simulink model "Target_Control_System"  (R2021b)
settings: Solver=FixedStepDiscrete  StartTime=0.0  StopTime=5  RelTol=1e-3
PreLoadFcn:
  | RTWConfigurationCB('preloadfcn', bdroot);
PostLoadFcn:
  | load('configuration/data_struct.mat');
  | load('configuration/fluxMaps_propMotor.mat');
  | load('configuration/parameterInit_PROP.mat');
  | load('configuration/parameterInit_PUMP.mat');
  | load('configuration/parameterInit_PITCH.mat');
  | load('configuration/parameterInit_TILT.mat');
  | %load('configuration/base_workspace_signal_definition.mat');
  | %load('resolvedatastores_to_baseworkspace_for_faster_simulation.mat');
model workspace (MAT data in the model file):
  SIMULATION_OPTIONS : Simulink.Parameter (value not decoded)
  TARGET_CODE_GEN : Simulink.Parameter (value not decoded)
  TCS_SAMPLE_FREQ_HZ : Simulink.Parameter (value not decoded)
symbols that are objects in the model workspace (value not decoded): TARGET_CODE_GEN, TCS_SAMPLE_FREQ_HZ
undefined symbols (not defined in the file): A_DQ_REF_LPF_INIT__PITCH, A_DQ_REF_LPF_INIT__PROP, A_DQ_REF_LPF_INIT__PUMP, A_DQ_REF_LPF_INIT__TILT, A_OBSERVER_CONFIDENCE_INIT__PITCH, A_OBSERVER_CONFIDENCE_INIT__PROP, A_OBSERVER_CONFIDENCE_INIT__PUMP, A_OBSERVER_CONFIDENCE_INIT__TILT, ACTUATOR_MAX_ANGLE_TRIP__PITCH, ACTUATOR_MIN_ANGLE_TRIP__PITCH, ACTUATOR_POS_SENSOR_INV_DIRECTION__PITCH, ACTUATOR_POS_SENSOR_INV_DIRECTION__TILT, ACTUATOR_POS_SENSOR_OFFSET__PITCH, ACTUATOR_POS_SENSOR_OFFSET__TILT, ADC_scaler1_baseaddr_TILT, ADC_SCALER_FLOAT_TO_FIXPOINT_EXPANSION, ANGLE_ELEC_FROM_SENSOR_OFFSET_INIT__PITCH, ANGLE_ELEC_FROM_SENSOR_OFFSET_INIT__PROP, ANGLE_ELEC_FROM_SENSOR_OFFSET_INIT__PUMP, ANGLE_ELEC_FROM_SENSOR_OFFSET_INIT__TILT, AUTO_CLEAR_FAULTS_ENABLED__PITCH, AUTO_CLEAR_FAULTS_ENABLED__PROP, AUTO_CLEAR_FAULTS_ENABLED__PUMP, AUTO_CLEAR_FAULTS_ENABLED__TILT, AUTO_CLEAR_FAULTS_WAIT_TICKS__PITCH, AUTO_CLEAR_FAULTS_WAIT_TICKS__PROP, AUTO_CLEAR_FAULTS_WAIT_TICKS__PUMP, AUTO_CLEAR_FAULTS_WAIT_TICKS__TILT, AUTO_I_ZERO_IDLE_TICKS__PITCH, AUTO_I_ZERO_IDLE_TICKS__PROP, AUTO_I_ZERO_IDLE_TICKS__PUMP, AUTO_I_ZERO_IDLE_TICKS__TILT, AUTO_I_ZERO_OFFSET_IDC_THRESHOLD__PITCH, AUTO_I_ZERO_OFFSET_IDC_THRESHOLD__PROP, AUTO_I_ZERO_OFFSET_IDC_THRESHOLD__PUMP, AUTO_I_ZERO_OFFSET_IDC_THRESHOLD__TILT, AUTO_I_ZERO_OFFSET_IPH_THRESHOLD__PITCH, AUTO_I_ZERO_OFFSET_IPH_THRESHOLD__PROP, AUTO_I_ZERO_OFFSET_IPH_THRESHOLD__PUMP, AUTO_I_ZERO_OFFSET_IPH_THRESHOLD__TILT, AUTO_SENSORLESS_SWITCHOVER_DISABLE_OMEGA, AUTO_SENSORLESS_SWITCHOVER_ENABLE_OMEGA, AUTO_SENSORLESS_SWITCHOVER_MIN_CONFIDENCE, AUXILIARY_PROTECTION_UNIT_BASEADDR__TILT, blanking_max_error_omega_INIT_PITCH, blanking_max_error_omega_INIT_TILT, blanking_max_error_position_INIT_PITCH, blanking_max_error_position_INIT_TILT, BRUTE_START_I_Q_REF_RAMP_SPEED__PITCH, BRUTE_START_I_Q_REF_RAMP_SPEED__PROP, BRUTE_START_I_Q_REF_RAMP_SPEED__PUMP, BRUTE_START_I_Q_REF_RAMP_SPEED__TILT, CONTROL_LOOP_DT_INIT__PITCH, CONTROL_LOOP_DT_INIT__PROP, CONTROL_LOOP_DT_INIT__PUMP, CONTROL_LOOP_DT_INIT__TILT, CORRECTION_FILTER_SCALE__PITCH, CORRECTION_FILTER_SCALE__PROP, CORRECTION_FILTER_SCALE__PUMP, CORRECTION_FILTER_SCALE__TILT ... (+458)
libraries: simulink x178, Reusables_Lib x24
(part 47 of 47)

== stateflow chart Target_Control_System/MainLoop/propMotor_mainLoop/motorTaskMainFastStep(&oProp)/enableDrive(&oProp) ==
  state Disabled
    state Default
    state Disable_Drive
      entry:
      oProp.oMot_.oState_.uiDriveState_ = 100;
      oProp.oMot_.oOut_.uiEnableGateDrive_ = 0x0;
      oProp.oMot_.oOut_.uiCurrentControllerActive_ = 0;
    state Simulation
      entry:
      oProp.oMot_.oState_.uiDriveState_ = 101;
      oProp.oMot_.oOut_.uiEnableGateDrive_ = 0x0;
    (default) -> (junction 391)
    (junction 391) -> Default [order 3]
    (junction 391) -> Disable_Drive [order 2] : [oProp.oMot_.oState_.uiDriveState_ >= 200 && ....
        |  oProp.oMot_.oState_.uiDriveState_ <= 299]
    (junction 391) -> Simulation [order 1] : [TARGET_CODE_GEN ==0]
  state Position_hold_mode
    // Mostly intended for the VP. In position hold mode, the inverter will inject 0 RPM current in the motor to passively hold a motor in place.
    // The position sensors are not needed for this.
    // When issuing the enable command, the drive enters state 226, which is just for flagging, the inverters do not actually turn on.
    // (Use a special command for that.)
    entry:
    oProp.oMot_.oState_.uiDriveState_ = 226;
    oProp.oIsr_.oParam_.oPiDataIq_.fState_ = 0;
    oProp.oIsr_.oParam_.oPiDataId_.fState_ = 0;
    // Pre-set 50% duty
    oProp.oMot_.oOut_.uiPwmRequestFromMain_ = 1;
    oProp.oMot_.oOut_.uiPwmDutyTicksFromMainA_ = uint32((oProp.oMot_.oParam_.fPwmPeriodTicksMainloopFloat_)/2);
    oProp.oMot_.oOut_.uiPwmDutyTicksFromMainB_ = uint32((oProp.oMot_.oParam_.fPwmPeriodTicksMainloopFloat_)/2);
    oProp.oMot_.oOut_.uiPwmDutyTicksFromMainC_ = uint32((oProp.oMot_.oParam_.fPwmPeriodTicksMainloopFloat_)/2);
  state DC_undervoltage_trip
    state Fault_A
      entry:
      oProp.oMot_.oOut_.uiCurrentControllerActive_ = 0;
      oProp.oMot_.oOut_.uiEnableGateDrive_ = 0;
    state Fault_B
      // If we were already in a fault state, store the previous fault:
      entry:
      oProp.oMot_.oOut_.uiLastFaultState_ = oProp.oMot_.oState_.uiDriveState_;
    state Fault_C
      entry:
      oProp.oMot_.oState_.uiDriveState_ = 1003;
    (default) -> (junction 164)
    (junction 164) -> Fault_A [order 1] : [oProp.oMot_.oState_.uiDriveState_>= 200]
    (junction 164) -> Fault_C [order 3]
    (junction 164) -> Fault_B [order 2] : [oProp.oMot_.oState_.uiDriveState_>= 1000]
    Fault_A -> Fault_B [order 1] : [oProp.oMot_.oState_.uiDriveState_>= 1000]
    Fault_A -> Fault_C [order 2]
    Fault_B -> Fault_C
  state Slave_start
    // Slave start is not applicable to position control.
    // Not a position control inverter; slave role is set: Perform a slave start (wait for the motor to 'somehow' reach a minimum speed, then jump on).
    entry:
    // We have to set one item aside; the desired rotation direction, as signalled by the sign of the current
    oProp.oMot_.oState_.fForcedAngleStartDirection_ = single(oProp.oMot_.oIn_.fIqSetpoint_ >= 0);
    // Don't actually turn on the output stage, but instead, monitor the motor feedback.
    // Once confident, perform a running start.
    // The rest is handled via state machine.
    oProp.oMot_.oState_.uiDriveState_ = 220;
  state setupForFlyingStart
    entry:
    oProp.oMot_.oOut_.uiPwmDutyTicksFromMainA_ = uint32((oProp.oMot_.oParam_.fPwmPeriodTicksMainloopFloat_)/2);
    oProp.oMot_.oOut_.uiPwmDutyTicksFromMainB_ = uint32((oProp.oMot_.oParam_.fPwmPeriodTicksMainloopFloat_)/2);
    oProp.oMot_.oOut_.uiPwmDutyTicksFromMainC_ = uint32((oProp.oMot_.oParam_.fPwmPeriodTicksMainloopFloat_)/2);
    oProp.oMot_.oState_.oRampDataOmegaERef_.fRampOut_ = oProp.oMot_.oIn_.fOmegaEObserverLpf2_;
    oProp.oMot_.oState_.oRampDataIqRef_.fRampOut_ = 0.0;
    oProp.oIsr_.oParam_.oPiDataIq_.fState_ = 0.0F;
    oProp.oIsr_.oParam_.oPiDataId_.fState_ = 0.0F;
    oProp.oMot_.oParam_.oPiDataRpm_.fState_ = 0.0F;
    oProp.oMot_.oParam_.oPid2DataRpmCtrl_.fState_ = 0.0F;
    oProp.oMot_.oState_.uiDriveState_ = 200;
    oProp.oIsr_.oState_.fOverspeedProtectionScaler_ = 1.0;
    oProp.oMot_.oState_.oPosSensor_.iAngleElecFromSensorNumOfIdenticalValues_ = 0;
    // release gate signals
    oProp.oMot_.oOut_.uiEnableGateDrive_ = 0x7;
    // Release control in main interrupt
    oProp.oMot_.oOut_.uiCurrentControllerActive_ = 1;
    // [SZ]: add automatic fan control here
  state Enabled
    // [SZ]: Still need to model the setupForFlyingStart() function, which involves calling NEON sin/cos functions in Stateflow
    state Open_loop_start
      // Open loop start from standstill. Risky, and rough on hardware
      state Open_loop_start_A
        entry:
        oProp.oMot_.oState_.oRampDataFluxFeedforwardGain_.fRampOut_ = 0.0;
        oProp.oMot_.oState_.oRampDataOmegaERef_.fRampOut_ = 0.0;
        oProp.oMot_.oState_.oRampDataIqRef_.fRampOut_ = 0.0;
        oProp.oMot_.oState_.uiDriveState_ = 200;
      state Open_loop_start_B
        entry:
        oProp.oMot_.oState_.uiDriveState_ = 205;
      (default) -> Open_loop_start_A
      Open_loop_start_A -> Open_loop_start_B [order 1] : [oProp.oMot_.oParam_.uiAutomaticFanControlMode_ == 1]
    state Standing_start
      // ----- Set up for forced angle start ----
      state Store_reference
        // Store original references and ramp rates aside:
        entry:
        oProp.oMot_.oState_.fForcedAngleStartOrigIRamp_ = oProp.oMot_.oState_.oRampDataIqRef_.oParam_.fUpslope_;
        // TODO: whatabout downslope?
        oProp.oMot_.oState_.fForcedAngleStartOrigOmega_ = oProp.oMot_.oState_.oRampDataOmegaERef_.fSetpoint_;
        oProp.oMot_.oState_.fForcedAngleStartOrigOmegaRamp_ = oProp.oMot_.oState_.oRampDataOmegaERef_.oParam_.fUpslope_;
        // The downslope is never touched, as it doesn't matter for forced angle start
        oProp.oMot_.oState_.uiForcedAngleStartOrigSpeedControllerActive_ = oProp.oMot_.oState_.uiSpeedControllerActive_;
        // We have to set one item aside; the desired rotation direction, as signalled by the sign of the current
        oProp.oMot_.oState_.fForcedAngleStartDirection_ = single(oProp.oMot_.oIn_.fIqSetpoint_ >= 0);
      state Global_signal
        // Signals to the rest of the program.
        oProp.oMot_.oOut_.uiForcedAngle_ = 1;
        oProp.oMot_.oState_.uiDriveState_ = 211;
      state Initialization
        // Set up initial values
        entry:
        oProp.oMot_.oState_.fIqRefBeforeRamp_ = oProp.oMot_.oParam_.fForcedAngleIRef_;
        oProp.oMot_.oState_.oRampDataIqRef_.oParam_.fUpslope_ = oProp.oMot_.oParam_.fForcedAngleIRamp_*10*(TARGET_CODE_GEN==0)+...
        oProp.oMot_.oParam_.fForcedAngleIRamp_*(TARGET_CODE_GEN==1); // Adjust for 100 Hz state machine in the simulation mode
        oProp.oMot_.oState_.oRampDataIqRef_.oParam_.fDownslope_ = oProp.oMot_.oState_.oRampDataIqRef_.oParam_.fUpslope_;
        oProp.oMot_.oState_.oRampDataOmegaERef_.oParam_.fUpslope_ = oProp.oMot_.oParam_.fForcedAngleOmegaERamp_*10*(TARGET_CODE_GEN==0)+...
        oProp.oMot_.oParam_.fForcedAngleOmegaERamp_*(TARGET_CODE_GEN==1); // Adjust for 100 Hz state machine in the simulation mode
        oProp.oMot_.oState_.oRampDataOmegaERef_.fRampOut_ = 0.0F;
        oProp.oMot_.oState_.oRampDataOmegaERef_.fSetpoint_ = 0.0F;
        oProp.oMot_.oState_.oRampDataIqRef_.fRampOut_ = 0.0F;
        oProp.oMot_.oState_.uiSpeedControllerActive_ = 0;
        oProp.oMot_.oState_.uiForcedAngleStartParametersSet_ = 1;
        oProp.oMot_.oState_.oRampDataFluxFeedforwardGain_.fRampOut_ = 0.0F;
      (default) -> Global_signal
      Global_signal -> (junction 233)
      (junction 233) -> Store_reference [order 1] : [!(oProp.oMot_.oState_.uiForcedAngleStartParametersSet_ == 1)]
      (junction 233) -> Initialization [order 2]
      Store_reference -> Initialization
    state Half_duty_preset
      // Pre-set 50% duty
      entry:
      oProp.oMot_.oOut_.uiPwmRequestFromMain_ = 1;
      oProp.oMot_.oOut_.uiPwmDutyTicksFromMainA_ = uint32((oProp.oMot_.oParam_.fPwmPeriodTicksMainloopFloat_)/2);
      oProp.oMot_.oOut_.uiPwmDutyTicksFromMainB_ = uint32((oProp.oMot_.oParam_.fPwmPeriodTicksMainloopFloat_)/2);
      oProp.oMot_.oOut_.uiPwmDutyTicksFromMainC_ = uint32((oProp.oMot_.oParam_.fPwmPeriodTicksMainloopFloat_)/2);
      oProp.oIsr_.oParam_.oPiDataIq_.fState_ = 0.0F;
      oProp.oIsr_.oParam_.oPiDataId_.fState_ = 0.0F;
      oProp.oMot_.oParam_.oPiDataRpm_.fState_ = 0.0F;
      oProp.oMot_.oParam_.oPid2DataRpmCtrl_.fState_ = 0.0F;
      oProp.oMot_.oState_.oPosSensor_.oPidDataPosCtrl_.fState_ = 0.0F;
      oProp.oMot_.oState_.oRampDataPos_.fRampOut_ = oProp.oMot_.oState_.oPosSensor_.oGbx_.fCurrentOutputAngle_;
      // Prevent jerk motions on start up.
      // [SZ]: Moved here to avoid the "Unconditional Path Out of State with During Actions or Child States" warning
    state Release_gate_signal
      entry:
      oProp.oIsr_.oState_.fOverspeedProtectionScaler_ = 1.0;
      oProp.oMot_.oState_.oPosSensor_.iAngleElecFromSensorNumOfIdenticalValues_ = 0;
      // release gate signals
      oProp.oMot_.oOut_.uiEnableGateDrive_ = 0x7;
      oProp.oMot_.oOut_.uiCurrentControllerActive_ = 1; // Release control in main interrupt
    (default) -> (junction 184)
    (junction 184) -> Open_loop_start [order 2]
    (junction 184) -> Standing_start [order 1] : [oProp.oMot_.oState_.uiForcedAngleStart_ == 1]
    Open_loop_start_A -> Half_duty_preset [order 2]
    Open_loop_start_B -> Half_duty_preset
    Initialization -> Half_duty_preset
    Half_duty_preset -> Release_gate_signal
  (default) -> Disabled
  Slave_start -> Disabled : [!(oProp.oMot_.oOut_.uiEnable_ == 1)]
  Position_hold_mode -> Disabled : [!(oProp.oMot_.oOut_.uiEnable_ == 1)]
  (junction 192) -> Disabled [order 1] : [oProp.oMot_.oState_.uiDriveState_ < 101 || oProp.oMot_.oState_.uiDriveState_ > 104 || !(oProp.oMot_.oOut_.uiEnable_ == 1)]
  Disabled -> (junction 192) : [oProp.oMot_.oOut_.uiEnable_ == 1]
  DC_undervoltage_trip -> Disabled : [oProp.oMot_.oOut_.fUdcLpf_>oProp.oMot_.oParam_.fUdcMinTrip_ || !(oProp.oMot_.oOut_.uiEnable_ == 1)]
  setupForFlyingStart -> Disabled : [!(oProp.oMot_.oOut_.uiEnable_ == 1)]
  Enabled -> Disabled : [!(oProp.oMot_.oOut_.uiEnable_ == 1)]
  (junction 192) -> Position_hold_mode [order 3] : [oProp.oMot_.oParam_.iForcedPositionHoldMode_ == 1]
  (junction 192) -> DC_undervoltage_trip [order 2] : [oProp.oMot_.oOut_.fUdcLpf_<oProp.oMot_.oParam_.fUdcMinTrip_]
  (junction 192) -> Slave_start [order 4] : [oProp.oMot_.oParam_.uiSlaveRole_ == 1 && !(oProp.oMot_.oState_.oPosSensor_.iPosControlEnabled_ == 1)]
  (junction 192) -> (junction 258) [order 5]
  (junction 258) -> setupForFlyingStart [order 2]
  (junction 258) -> Enabled [order 1] : [oProp.oMot_.oState_.uiDriveState_ == 101 || oProp.oMot_.oState_.uiDriveState_ == 103]
  data: oProp data_store_memory; TARGET_CODE_GEN parameter

== stateflow chart Target_Control_System/MainLoop/pumpMotor_mainLoop/motorTaskMainFastStep(&oPump)/enableDrive(&oPump) ==
  state Disabled
    state Default
    state Disable_Drive
      entry:
      oPump.oMot_.oState_.uiDriveState_ = 100;
      oPump.oMot_.oOut_.uiEnableGateDrive_ = 0x0;
      oPump.oMot_.oOut_.uiCurrentControllerActive_ = 0;
    state Simulation
      entry:
      oPump.oMot_.oState_.uiDriveState_ = 101;
      oPump.oMot_.oOut_.uiEnableGateDrive_ = 0x0;
    (default) -> (junction 264)
    (junction 264) -> Default [order 3]
    (junction 264) -> Disable_Drive [order 2] : [oPump.oMot_.oState_.uiDriveState_ >= 200 && ....
        |  oPump.oMot_.oState_.uiDriveState_ <= 299]
    (junction 264) -> Simulation [order 1] : [TARGET_CODE_GEN ==0]
  state Position_hold_mode
    // Mostly intended for the VP. In position hold mode, the inverter will inject 0 RPM current in the motor to passively hold a motor in place.
    // The position sensors are not needed for this.
    // When issuing the enable command, the drive enters state 226, which is just for flagging, the inverters do not actually turn on.
    // (Use a special command for that.)
    entry:
    oPump.oMot_.oState_.uiDriveState_ = 226;
    oPump.oIsr_.oParam_.oPiDataIq_.fState_ = 0;
    oPump.oIsr_.oParam_.oPiDataId_.fState_ = 0;
    // Pre-set 50% duty
    oPump.oMot_.oOut_.uiPwmRequestFromMain_ = 1;
    oPump.oMot_.oOut_.uiPwmDutyTicksFromMainA_ = uint32((oPump.oMot_.oParam_.fPwmPeriodTicksMainloopFloat_)/2);
    oPump.oMot_.oOut_.uiPwmDutyTicksFromMainB_ = uint32((oPump.oMot_.oParam_.fPwmPeriodTicksMainloopFloat_)/2);
    oPump.oMot_.oOut_.uiPwmDutyTicksFromMainC_ = uint32((oPump.oMot_.oParam_.fPwmPeriodTicksMainloopFloat_)/2);
  state DC_undervoltage_trip
    state Fault_A
      entry:
      oPump.oMot_.oOut_.uiCurrentControllerActive_ = 0;
      oPump.oMot_.oOut_.uiEnableGateDrive_ = 0;
    state Fault_B
      // If we were already in a fault state, store the previous fault:
      entry:
      oPump.oMot_.oOut_.uiLastFaultState_ = oPump.oMot_.oState_.uiDriveState_;
    state Fault_C
      entry:
      oPump.oMot_.oState_.uiDriveState_ = 1003;
    (default) -> (junction 164)
    (junction 164) -> Fault_A [order 1] : [oPump.oMot_.oState_.uiDriveState_>= 200]
    (junction 164) -> Fault_C [order 3]
    (junction 164) -> Fault_B [order 2] : [oPump.oMot_.oState_.uiDriveState_>= 1000]
    Fault_A -> Fault_B [order 1] : [oPump.oMot_.oState_.uiDriveState_>= 1000]
    Fault_A -> Fault_C [order 2]
    Fault_B -> Fault_C
  state Slave_start
    // Slave start is not applicable to position control.
    // Not a position control inverter; slave role is set: Perform a slave start (wait for the motor to 'somehow' reach a minimum speed, then jump on).
    entry:
    // We have to set one item aside; the desired rotation direction, as signalled by the sign of the current
    oPump.oMot_.oState_.fForcedAngleStartDirection_ = single(oPump.oMot_.oIn_.fIqSetpoint_ >= 0);
    // in other areas of MBD, we use oPump.oMot_.oState_.oRampDataIqRef_.fRampOut_...should we here?
    // Don't actually turn on the output stage, but instead, monitor the motor feedback.
    // Once confident, perform a running start.
    // The rest is handled via state machine.
    oPump.oMot_.oState_.uiDriveState_ = 220;
  state setupForFlyingStart
    entry:
    oPump.oMot_.oOut_.uiPwmDutyTicksFromMainA_ = uint32((oPump.oMot_.oParam_.fPwmPeriodTicksMainloopFloat_)/2);
    oPump.oMot_.oOut_.uiPwmDutyTicksFromMainB_ = uint32((oPump.oMot_.oParam_.fPwmPeriodTicksMainloopFloat_)/2);
    oPump.oMot_.oOut_.uiPwmDutyTicksFromMainC_ = uint32((oPump.oMot_.oParam_.fPwmPeriodTicksMainloopFloat_)/2);
    oPump.oMot_.oState_.oRampDataOmegaERef_.fRampOut_ = oPump.oMot_.oIn_.fOmegaEObserverLpf2_;
    oPump.oMot_.oState_.oRampDataIqRef_.fRampOut_ = 0.0;
    oPump.oIsr_.oParam_.oPiDataIq_.fState_ = 0.0F;
    oPump.oIsr_.oParam_.oPiDataId_.fState_ = 0.0F;
    oPump.oMot_.oParam_.oPiDataRpm_.fState_ = 0.0F;
    oPump.oMot_.oParam_.oPid2DataRpmCtrl_.fState_ = 0.0F;
    oPump.oMot_.oState_.uiDriveState_ = 200;
    oPump.oIsr_.oState_.fOverspeedProtectionScaler_ = 1.0;
    oPump.oMot_.oState_.oPosSensor_.iAngleElecFromSensorNumOfIdenticalValues_ = 0;
    // release gate signals
    oPump.oMot_.oOut_.uiEnableGateDrive_ = 0x7;
    // Release control in main interrupt
    oPump.oMot_.oOut_.uiCurrentControllerActive_ = 1;
  state Automatic_Fan
    entry:
    oPump.oMot_.oState_.uiDriveState_ = 205;
  state Enabled
    // [SZ]: Still need to model the setupForFlyingStart() function, which involves calling NEON sin/cos functions in Stateflow
    state Open_loop_start
      // Open loop start from standstill. Risky, and rough on hardware
      state Open_loop_start_A
        entry:
        oPump.oMot_.oState_.oRampDataFluxFeedforwardGain_.fRampOut_ = 0.0;
        oPump.oMot_.oState_.oRampDataOmegaERef_.fRampOut_ = 0.0;
        oPump.oMot_.oState_.oRampDataIqRef_.fRampOut_ = 0.0;
        oPump.oMot_.oState_.uiDriveState_ = 200;
      state Automatic_Fan
        entry:
        oPump.oMot_.oState_.uiDriveState_ = 205;
      (default) -> Open_loop_start_A
      Open_loop_start_A -> Enabled.Open_loop_start.Automatic_Fan [order 1] : [oPump.oMot_.oParam_.uiAutomaticFanControlMode_ == 1]
    state Standing_start
      // ----- Set up for forced angle start ----
      state Store_reference
        // Store original references and ramp rates aside:
        entry:
        oPump.oMot_.oState_.fForcedAngleStartOrigIRamp_ = oPump.oMot_.oState_.oRampDataIqRef_.oParam_.fUpslope_;
        // TODO: whatabout downslope?
        oPump.oMot_.oState_.fForcedAngleStartOrigOmega_ = oPump.oMot_.oState_.oRampDataOmegaERef_.fSetpoint_;
        oPump.oMot_.oState_.fForcedAngleStartOrigOmegaRamp_ = oPump.oMot_.oState_.oRampDataOmegaERef_.oParam_.fUpslope_;
        // The downslope is never touched, as it doesn't matter for forced angle start
        oPump.oMot_.oState_.uiForcedAngleStartOrigSpeedControllerActive_ = oPump.oMot_.oState_.uiSpeedControllerActive_;
        // We have to set one item aside; the desired rotation direction, as signalled by the sign of the current
        oPump.oMot_.oState_.fForcedAngleStartDirection_ = single(oPump.oMot_.oIn_.fIqSetpoint_ >= 0);
      state Global_signal
        // Signals to the rest of the program.
        oPump.oMot_.oOut_.uiForcedAngle_ = 1;
        oPump.oMot_.oState_.uiDriveState_ = 211;
      state Initialization
        // Set up initial values
        entry:
        oPump.oMot_.oState_.fIqRefBeforeRamp_ = oPump.oMot_.oParam_.fForcedAngleIRef_;
        oPump.oMot_.oState_.oRampDataIqRef_.oParam_.fUpslope_ = oPump.oMot_.oParam_.fForcedAngleIRamp_*10*(TARGET_CODE_GEN==0)+...
        oPump.oMot_.oParam_.fForcedAngleIRamp_*(TARGET_CODE_GEN==1); // Adjust for 100 Hz state machine
        oPump.oMot_.oState_.oRampDataIqRef_.oParam_.fDownslope_ = oPump.oMot_.oState_.oRampDataIqRef_.oParam_.fUpslope_;
        oPump.oMot_.oState_.oRampDataOmegaERef_.oParam_.fUpslope_ = oPump.oMot_.oParam_.fForcedAngleOmegaERamp_*10*(TARGET_CODE_GEN==0)+...
        oPump.oMot_.oParam_.fForcedAngleOmegaERamp_*(TARGET_CODE_GEN==1); // Adjust for 100 Hz state machine
        oPump.oMot_.oState_.oRampDataOmegaERef_.fRampOut_ = 0.0F;
        oPump.oMot_.oState_.oRampDataOmegaERef_.fSetpoint_ = 0.0F;
        oPump.oMot_.oState_.oRampDataIqRef_.fRampOut_ = 0.0F;
        oPump.oMot_.oState_.uiSpeedControllerActive_ = 0;
        oPump.oMot_.oState_.uiForcedAngleStartParametersSet_ = 1;
        oPump.oMot_.oState_.oRampDataFluxFeedforwardGain_.fRampOut_ = 0.0F;
      (default) -> Global_signal
      Global_signal -> (junction 233)
      (junction 233) -> Store_reference [order 1] : [!(oPump.oMot_.oState_.uiForcedAngleStartParametersSet_ == 1)]
      (junction 233) -> Initialization [order 2]
      Store_reference -> Initialization
    state Half_duty_preset
      // Pre-set 50% duty
      entry:
      oPump.oMot_.oOut_.uiPwmRequestFromMain_ = 1;
      oPump.oMot_.oOut_.uiPwmDutyTicksFromMainA_ = uint32((oPump.oMot_.oParam_.fPwmPeriodTicksMainloopFloat_)/2);
      oPump.oMot_.oOut_.uiPwmDutyTicksFromMainB_ = uint32((oPump.oMot_.oParam_.fPwmPeriodTicksMainloopFloat_)/2);
      oPump.oMot_.oOut_.uiPwmDutyTicksFromMainC_ = uint32((oPump.oMot_.oParam_.fPwmPeriodTicksMainloopFloat_)/2);
      oPump.oIsr_.oParam_.oPiDataIq_.fState_ = 0.0F;
      oPump.oIsr_.oParam_.oPiDataId_.fState_ = 0.0F;
      oPump.oMot_.oParam_.oPiDataRpm_.fState_ = 0.0F;
      oPump.oMot_.oParam_.oPid2DataRpmCtrl_.fState_ = 0.0F;
      oPump.oMot_.oState_.oPosSensor_.oPidDataPosCtrl_.fState_ = 0.0F;
      oPump.oMot_.oState_.oRampDataPos_.fRampOut_ = oPump.oMot_.oState_.oPosSensor_.oGbx_.fCurrentOutputAngle_;
      // Prevent jerk motions on start up.
      // [SZ]: Moved here to avoid the "Unconditional Path Out of State with During Actions or Child States" warning
    state Release_gate_signal
      entry:
      oPump.oIsr_.oState_.fOverspeedProtectionScaler_ = 1.0;
      oPump.oMot_.oState_.oPosSensor_.iAngleElecFromSensorNumOfIdenticalValues_ = 0;
      // release gate signals
      oPump.oMot_.oOut_.uiEnableGateDrive_ = 0x7;
      oPump.oMot_.oOut_.uiCurrentControllerActive_ = 1; // Release control in main interrupt
    (default) -> (junction 184)
    (junction 184) -> Open_loop_start [order 2]
    (junction 184) -> Standing_start [order 1] : [oPump.oMot_.oState_.uiForcedAngleStart_ == 1]
    Open_loop_start_A -> Half_duty_preset [order 2]
    Enabled.Open_loop_start.Automatic_Fan -> Half_duty_preset
    Initialization -> Half_duty_preset
    Half_duty_preset -> Release_gate_signal
  (default) -> Disabled
  Slave_start -> Disabled : [!(oPump.oMot_.oOut_.uiEnable_ == 1)]
  Position_hold_mode -> Disabled : [!(oPump.oMot_.oOut_.uiEnable_ == 1)]
  (junction 192) -> Disabled [order 1] : [oPump.oMot_.oState_.uiDriveState_ < 101 || oPump.oMot_.oState_.uiDriveState_ > 104 ...
      |  || !(oPump.oMot_.oOut_.uiEnable_ == 1)]
  Disabled -> (junction 192) : [oPump.oMot_.oOut_.uiEnable_ == 1]
  DC_undervoltage_trip -> Disabled : [oPump.oMot_.oOut_.fUdcLpf_>oPump.oMot_.oParam_.fUdcMinTrip_ || !(oPump.oMot_.oOut_.uiEnable_ == 1)]
  (junction 261) -> Disabled : [!(oPump.oMot_.oOut_.uiEnable_ == 1)]
  Enabled -> Disabled : [!(oPump.oMot_.oOut_.uiEnable_ == 1)]
  (junction 192) -> Position_hold_mode [order 3] : [oPump.oMot_.oParam_.iForcedPositionHoldMode_ == 1]
  (junction 192) -> DC_undervoltage_trip [order 2] : [oPump.oMot_.oOut_.fUdcLpf_<oPump.oMot_.oParam_.fUdcMinTrip_]
  (junction 192) -> Slave_start [order 4] : [oPump.oMot_.oParam_.uiSlaveRole_ == 1 && !(oPump.oMot_.oState_.oPosSensor_.iPosControlEnabled_ == 1)]
  (junction 192) -> (junction 254) [order 5]
  (junction 254) -> setupForFlyingStart [order 2]
  (junction 254) -> Enabled [order 1] : [oPump.oMot_.oState_.uiDriveState_ == 101 || oPump.oMot_.oState_.uiDriveState_ == 103]
  setupForFlyingStart -> (junction 261) [order 2]
  Automatic_Fan -> (junction 261)
  setupForFlyingStart -> Automatic_Fan [order 1] : [oPump.oMot_.oParam_.uiAutomaticFanControlMode_ == 1]
  data: oPump data_store_memory; TARGET_CODE_GEN parameter
